simulink model "A4_Feder_Masse_Schwinger"  (R2016a)
settings: Solver=ode1  StartTime=0.0  StopTime=100  FixedStep=0.00001  RelTol=1e-3
settings Model: Creator=Michaél  LastModifiedBy=Michaél

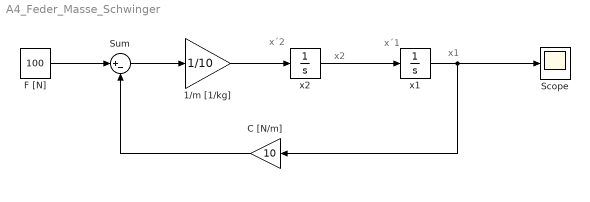
== system A4_Feder_Masse_Schwinger ==
  note: x´2
  note: x2
  note: x´1
  note: x1
  1/m [1/kg] : Gain  Gain=1/10
  C [N/m] : Gain  Gain=10
  F [N] : Constant  Value=100
  Scope : Scope
  Sum : Sum  Inputs=|+-
  x1 : Integrator
  x2 : Integrator
  wires:
  1/m [1/kg]/1 -> x2/1
  x2/1 -> x1/1
  Sum/1 -> 1/m [1/kg]/1
  F [N]/1 -> Sum/1
  x1/1 -> Scope/1, C [N/m]/1
  C [N/m]/1 -> Sum/2
